simulink model "MotorIdent"  (R2013a)
settings: Solver=FixedStepDiscrete  StartTime=0.0  StopTime=60  FixedStep=0.01  RelTol=1e-3
values from neighbouring files (symbols this model uses):
  joint = CoupledJoints('experiments', 'iCubGenova03', 'torso')    [CoupledExper-IDLE.m]    (also in CoupledExper.m = joint.loadRefFile('ref'); CoupledJoints.m = [joint Motor(date,robotName, part, type,'yaw')]; JointStructure.m = struct; ReferenceLoad.m = joint.loadReference('ref'))
  Reference = struct    [CoupledJoints.m]    (also in ReferenceLoad.m; WBLMotor.m)
libraries: WBCLibrary x12
settings Model: Creator=Raffaello  LastModifiedBy=Raffaello
settings DataIOCC: LimitDataPoints=off  OutputSaveName=out

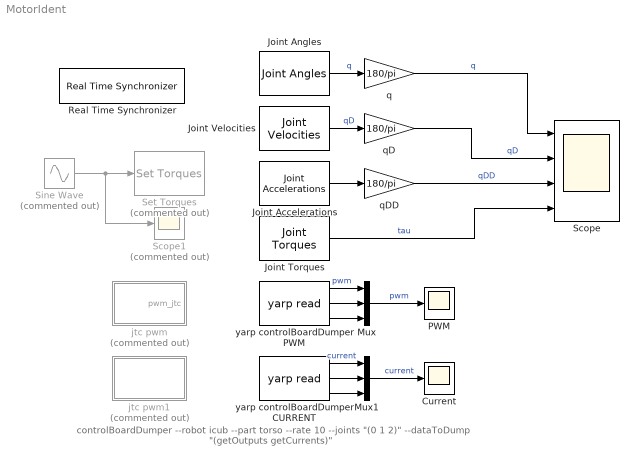
== system MotorIdent ==
  note: controlBoardDumper --robot icub --part torso --rate 10 --joints "(0 1 2)" --dataToDump "(getOutputs getCurrents)"
  Current : Scope
      settings: YMin=-3750  YMax=1750  SaveName=ScopeData3
  Joint Accelerations : WBCLibrary/wholeBodyStates/Joint Accelerations  robotName=robotName  localName=localName
  Joint Angles : WBCLibrary/wholeBodyStates/Joint Angles  robotName=robotName  localName=localName
  Joint Torques : WBCLibrary/wholeBodyStates/Joint Torques  robotName=robotName  localName=localName
  Joint Velocities : WBCLibrary/wholeBodyStates/Joint Velocities  robotName=robotName  localName=localName
  Mux : Mux  Inputs=3
  Mux1 : Mux  Inputs=3
  PWM : Scope
      settings: TimeRange=60  YMin=-80  YMax=80
  Real Time Synchronizer : WBCLibrary/Utilities/Real Time Synchronizer  Priority=-10  threadPeriod=Ts
  Scope : Scope  NumInputPorts=4
      settings: ShowLegends=on  TimeRange=60  YMin=-60~-40~-150~-10  YMax=40~60~150~10  SaveName=ScopeData2
  Scope1 : Scope  Commented=on
      settings: SaveName=ScopeData4
  Set Torques : WBCLibrary/wholeBodyActuators/Set Torques  Commented=on  val=6  robotName=robotName  localName=localName
  Sine Wave : Sin  Commented=on  Amplitude=Reference.sinAmp  Bias=Reference.sinBias  Frequency=Reference.sinFreq*2*pi  SampleTime=0
  jtc pwm : Subsystem  Commented=on
  jtc pwm1 : Subsystem  Commented=on
  q : Gain  Gain=180/pi
  qD : Gain  Gain=180/pi
  qDD : Gain  Gain=180/pi
  yarp controlBoardDumper CURRENT : WBCLibrary/Utilities/yarp read  from=['/controlBoardDumper/' joint.group_select '/getCurrents']  to='...'  num=3  blocking=off  timestamp=off
  yarp controlBoardDumper PWM : WBCLibrary/Utilities/yarp read  from=['/controlBoardDumper/' joint.group_select '/getOutputs']  to='...'  num=3  blocking=off  timestamp=off
  wires:
  Sine Wave/1 -> Scope1/1, Set Torques/1
  Joint Angles/1 -> q/1  "q"
  Joint Velocities/1 -> qD/1  "qD"
  Joint Torques/1 -> Scope/4  "tau"
  q/1 -> Scope/1  "q"
  qD/1 -> Scope/2  "qD"
  Mux/1 -> PWM/1  "pwm"
  Mux1/1 -> Current/1  "current"
  Joint Accelerations/1 -> qDD/1
  qDD/1 -> Scope/3  "qDD"
  yarp controlBoardDumper PWM/1 -> Mux/1  "pwm"
  yarp controlBoardDumper PWM/2 -> Mux/2
  yarp controlBoardDumper PWM/3 -> Mux/3
  yarp controlBoardDumper CURRENT/1 -> Mux1/1  "current"
  yarp controlBoardDumper CURRENT/2 -> Mux1/2
  yarp controlBoardDumper CURRENT/3 -> Mux1/3

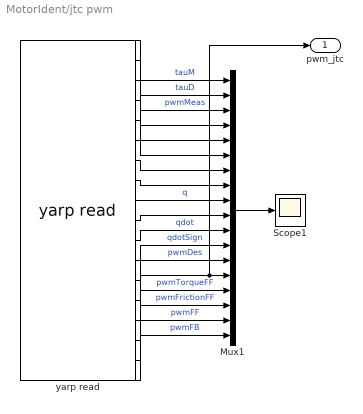
== system MotorIdent/jtc pwm ==
  Mux1 : Mux  Inputs=18
  Scope1 : Scope
      settings: ShowLegends=on
  yarp read : WBCLibrary/Utilities/yarp read  from=['/jtc/monitor:o']  to='...'  num=18  blocking=off  timestamp=off
  pwm_jtc : Outport
  wires:
  yarp read/18 -> Mux1/18  "pwmFB"
  Mux1/1 -> Scope1/1
  yarp read/1 -> Mux1/1  "tauM"
  yarp read/2 -> Mux1/2  "tauD"
  yarp read/3 -> Mux1/3
  yarp read/4 -> Mux1/4
  yarp read/5 -> Mux1/5
  yarp read/10 -> Mux1/10
  yarp read/6 -> Mux1/6
  yarp read/7 -> Mux1/7
  yarp read/8 -> Mux1/8
  yarp read/9 -> Mux1/9  "q"
  yarp read/11 -> Mux1/11  "qdot"
  yarp read/12 -> Mux1/12  "qdotSign"
  yarp read/13 -> Mux1/13  "pwmDes"
  yarp read/14 -> pwm_jtc/1, Mux1/14  "pwmMeas"
  yarp read/15 -> Mux1/15  "pwmTorqueFF"
  yarp read/16 -> Mux1/16  "pwmFrictionFF"
  yarp read/17 -> Mux1/17  "pwmFF"

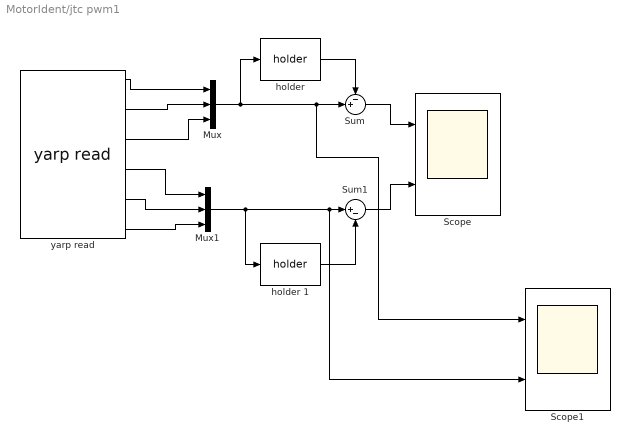
== system MotorIdent/jtc pwm1 ==
  Mux : Mux  Inputs=3
  Mux1 : Mux  Inputs=3
  Scope : Scope  NumInputPorts=2
      settings: ShowLegends=on  TimeRange=10  YMin=-12~-1.8  YMax=5~0.4  SaveName=ScopeData5
  Scope1 : Scope  NumInputPorts=2
      settings: ShowLegends=on  TimeRange=10  YMin=-20~-5.5  YMax=180~0.5  SaveName=ScopeData6
  Sum : Sum  Inputs=-+|
  Sum1 : Sum  Inputs=|+-
  "holder " : WBCLibrary/Utilities/holder 
  holder 1 : WBCLibrary/Utilities/holder 
  yarp read : WBCLibrary/Utilities/yarp read  from=['/icub/right_arm/analog:o']  to='...'  num=6  blocking=off  timestamp=off
  wires:
  Mux1/1 -> holder 1/1, Scope1/2, Sum1/1
  yarp read/1 -> Mux/1
  yarp read/2 -> Mux/2
  yarp read/3 -> Mux/3
  yarp read/4 -> Mux1/1
  yarp read/5 -> Mux1/2
  yarp read/6 -> Mux1/3
  Sum/1 -> Scope/1
  "holder "/1 -> Sum/1
  Sum1/1 -> Scope/2
  holder 1/1 -> Sum1/2
  Mux/1 -> Scope1/1, Sum/2, "holder "/1
